simulink model "MSDR_DH_DeplV1sim"  (R2019a)
settings: Solver=ode45  StartTime=0.0  StopTime=simtime  FixedStep=0.1  MaxStep=ts_max  RelTol=rel_tolerance
values from neighbouring files (symbols this model uses):
  a_f = 1E-5*depl_fuel_temp_coef(depl_index)    [MSDR_DH_DeplV1para.m]
  a_g = 1E-5*depl_grap_temp_coef(depl_index)    [MSDR_DH_DeplV1para.m]
  A_s = 1.2245    [MSDR_DH_DeplV1para.m]
  beta = depl_beta(depl_index,:)    [MSDR_DH_DeplV1para.m]
  beta_t = sum(beta)    [MSDR_DH_DeplV1para.m]
  Cp_f = depl_Cp_Fuel_coef*1.355616e-3    [MSDR_DH_DeplV1para.m]
  Cp_p = Cp_s_shx    [MSDR_DH_DeplV1para.m]
  Cp_s = Cp_s*1e-6    (= 3.588208e-09)    [MSDR_DH_DeplV1para.m]
  Cp_sc = 4761.392e-6    (= 0.004761392)    [MSDR_DH_DeplV1para.m]
  Cp_w = 456.056e-6    (= 0.000456056)    [MSDR_DH_DeplV1para.m]
  D_it = 0.0141478    [MSDR_DH_DeplV1para.m]
  D_ot = 0.015875    [MSDR_DH_DeplV1para.m]
  DHRS_TIME_K = 10    [MSDR_DH_DeplV1para.m]
  dHs_dPs = -0.042433622114357    (= -0.0424336221144)    [MSDR_DH_DeplV1para.m]
  Epsilon = 1E-3    (= 0.001)    [MSDR_DH_DeplV1para.m]
  Fiss_factor = 2.464783802008740e-03    (= 0.00246478380201)    [MSDR_DH_DeplV1para.m]
  gamma0 = 9.635981959409105e-01    (= 0.963598195941)    [MSDR_DH_DeplV1para.m]
  gamma1 = 3.560674858154914e-02    (= 0.0356067485815)    [MSDR_DH_DeplV1para.m]
  gamma2 = 7.950554775404400e-04    (= 0.00079505547754)    [MSDR_DH_DeplV1para.m]
  gamma_I = 5.1135e-2    (= 0.051135)    [MSDR_DH_DeplV1para.m]
  gamma_Pm = 1.08E-2    (= 0.0108)    [MSDR_DH_DeplV1para.m]
  gamma_Xe = 1.1628e-2    (= 0.011628)    [MSDR_DH_DeplV1para.m]
  h_pw = h_s_shx    [MSDR_DH_DeplV1para.m]
  h_wb = 13349.334646671E-6    (= 0.0133493346467)    [MSDR_DH_DeplV1para.m]
  h_ws = 5732.378387768E-6    (= 0.00573237838777)    [MSDR_DH_DeplV1para.m]
  h_wsc = 8385.005556375E-6    (= 0.00838500555638)    [MSDR_DH_DeplV1para.m]
  hA_fg = [h_fg*A_fg/2, h_fg*A_fg/2]    [MSDR_DH_DeplV1para.m]
  hA_p_phx1 = h_p_phx*A_p_phx    [MSDR_DH_DeplV1para.m]
  hA_p_phx2 = h_p_phx*A_p_phx    [MSDR_DH_DeplV1para.m]
  hA_p_phx3 = h_p_phx*A_p_phx    [MSDR_DH_DeplV1para.m]
  hA_p_phx4 = h_p_phx*A_p_phx    [MSDR_DH_DeplV1para.m]
  hA_p_phx5 = h_p_phx*A_p_phx    [MSDR_DH_DeplV1para.m]
  hA_p_phx6 = h_p_phx*A_p_phx    [MSDR_DH_DeplV1para.m]
  hA_p_shx1 = h_p_shx*A_p_shx    [MSDR_DH_DeplV1para.m]
  hA_p_shx2 = h_p_shx*A_p_shx    [MSDR_DH_DeplV1para.m]
  hA_p_shx3 = h_p_shx*A_p_shx    [MSDR_DH_DeplV1para.m]
  hA_p_shx4 = h_p_shx*A_p_shx    [MSDR_DH_DeplV1para.m]
  hA_p_shx5 = h_p_shx*A_p_shx    [MSDR_DH_DeplV1para.m]
  hA_p_shx6 = h_p_shx*A_p_shx    [MSDR_DH_DeplV1para.m]
  hA_s_phx1 = h_s_phx*A_s_phx    [MSDR_DH_DeplV1para.m]
  hA_s_phx2 = h_s_phx*A_s_phx    [MSDR_DH_DeplV1para.m]
  hA_s_phx3 = h_s_phx*A_s_phx    [MSDR_DH_DeplV1para.m]
  hA_s_phx4 = h_s_phx*A_s_phx    [MSDR_DH_DeplV1para.m]
  hA_s_phx5 = h_s_phx*A_s_phx    [MSDR_DH_DeplV1para.m]
  hA_s_phx6 = h_s_phx*A_s_phx    [MSDR_DH_DeplV1para.m]
  hA_s_shx1 = h_s_shx*A_s_shx    [MSDR_DH_DeplV1para.m]
  hA_s_shx2 = h_s_shx*A_s_shx    [MSDR_DH_DeplV1para.m]
  hA_s_shx3 = h_s_shx*A_s_shx    [MSDR_DH_DeplV1para.m]
  hA_s_shx4 = h_s_shx*A_s_shx    [MSDR_DH_DeplV1para.m]
  hA_s_shx5 = h_s_shx*A_s_shx    [MSDR_DH_DeplV1para.m]
  hA_s_shx6 = h_s_shx*A_s_shx    [MSDR_DH_DeplV1para.m]
  I_0 = gamma_I*Sig_f_msdr*phi_0/lam_I    [MSDR_DH_DeplV1para.m]
  Ifa = [0.25, 0.25]    [MSDR_DH_DeplV1para.m]
  Ifb = [0.25, 0.25]    [MSDR_DH_DeplV1para.m]
  Ig = [0.5, 0.5]    [MSDR_DH_DeplV1para.m]
  K_1 = 11.632248097704855    (= 11.6322480977)    [MSDR_DH_DeplV1para.m]
  K_4 = b(1)    [MSDR_DH_DeplV1para.m]
  K_5 = a(1)    [MSDR_DH_DeplV1para.m]
  K_b = 12.834854076292217    (= 12.8348540763)    [MSDR_DH_DeplV1para.m]
  K_pump = 1/5    (= 0.2)    [MSDR_DH_DeplV1para.m]
  K_sc = -17.615718797133468    (= -17.6157187971)    [MSDR_DH_DeplV1para.m]
  ka = [0.235, 0.235]    [MSDR_DH_DeplV1para.m]
  kb = [0.235, 0.235]    [MSDR_DH_DeplV1para.m]
  kga = [0.015, 0.015]    [MSDR_DH_DeplV1para.m]
  kgb = [0.015, 0.015]    [MSDR_DH_DeplV1para.m]
  L = 8.5344    [MSDR_DH_DeplV1para.m]
  L_b = 2.3645    [MSDR_DH_DeplV1para.m]
  L_s = 4.723    [MSDR_DH_DeplV1para.m]
  Lam = depl_Lam(depl_index)    [MSDR_DH_DeplV1para.m]
  lam = [1.240E-02, 3.05E-02, 1.11E-01, 3.01E-01, 1.140E+00, 3.014E+00]    [MSDR_DH_DeplV1para.m]
  lam_bubl = 2.0e-2    (= 0.02)    [MSDR_DH_DeplV1para.m]
  lam_I = 2.875e-5    (= 2.875e-05)    [MSDR_DH_DeplV1para.m]
  lam_Pm = log(2)/(2.21*24*3600)    [MSDR_DH_DeplV1para.m]
  lam_Xe = 2.0916e-5    (= 2.0916e-05)    [MSDR_DH_DeplV1para.m]
  lambda0 = 0.0945298    [MSDR_DH_DeplV1para.m]
  lambda1 = 0.00441957    [MSDR_DH_DeplV1para.m]
  lambda2 = 8.60979e-05    [MSDR_DH_DeplV1para.m]
  m_3m = W_3*2    (= 8618.207327)    [MSDR_DH_DeplV1para.m]
  m_f_t = total_mp_phx + core_fm + mp_phxm*3 + m_fm    [MSDR_DH_DeplV1para.m]
  m_fm = W_f*1    (= 4989.48)    [MSDR_DH_DeplV1para.m]
  M_stm = 0.018    [MSDR_DH_DeplV1para.m]
  mcp_fa = mfa*Cp_f    [MSDR_DH_DeplV1para.m]
  mcp_fb = mfb*Cp_f    [MSDR_DH_DeplV1para.m]
  mcp_g = mg*Cp_g    [MSDR_DH_DeplV1para.m]
  mcp_p_phx1 = Cp_p_phx*mp_phx1    [MSDR_DH_DeplV1para.m]
  mcp_p_phx2 = Cp_p_phx*mp_phx2    [MSDR_DH_DeplV1para.m]
  mcp_p_phx3 = Cp_p_phx*mp_phx3    [MSDR_DH_DeplV1para.m]
  mcp_p_phx4 = Cp_p_phx*mp_phx4    [MSDR_DH_DeplV1para.m]
  mcp_p_phx5 = Cp_p_phx*mp_phx5    [MSDR_DH_DeplV1para.m]
  mcp_p_phx6 = Cp_p_phx*mp_phx6    [MSDR_DH_DeplV1para.m]
  mcp_p_shx1 = Cp_p_shx*mp_shx1    [MSDR_DH_DeplV1para.m]
  mcp_p_shx2 = Cp_p_shx*mp_shx2    [MSDR_DH_DeplV1para.m]
  mcp_p_shx3 = Cp_p_shx*mp_shx3    [MSDR_DH_DeplV1para.m]
  mcp_p_shx4 = Cp_p_shx*mp_shx4    [MSDR_DH_DeplV1para.m]
  mcp_p_shx5 = Cp_p_shx*mp_shx5    [MSDR_DH_DeplV1para.m]
  mcp_p_shx6 = Cp_p_shx*mp_shx6    [MSDR_DH_DeplV1para.m]
  mcp_s_phx1 = Cp_s_phx*ms_phx1    [MSDR_DH_DeplV1para.m]
  mcp_s_phx2 = Cp_s_phx*ms_phx2    [MSDR_DH_DeplV1para.m]
  mcp_s_phx3 = Cp_s_phx*ms_phx3    [MSDR_DH_DeplV1para.m]
  mcp_s_phx4 = Cp_s_phx*ms_phx4    [MSDR_DH_DeplV1para.m]
  mcp_s_phx5 = Cp_s_phx*ms_phx5    [MSDR_DH_DeplV1para.m]
  mcp_s_phx6 = Cp_s_phx*ms_phx6    [MSDR_DH_DeplV1para.m]
  mcp_s_shx1 = Cp_s_shx*ms_shx1    [MSDR_DH_DeplV1para.m]
  mcp_s_shx2 = Cp_s_shx*ms_shx1    [MSDR_DH_DeplV1para.m]
  mcp_s_shx3 = Cp_s_shx*ms_shx1    [MSDR_DH_DeplV1para.m]
  mcp_s_shx4 = Cp_s_shx*ms_shx1    [MSDR_DH_DeplV1para.m]
  mcp_s_shx5 = Cp_s_shx*ms_shx1    [MSDR_DH_DeplV1para.m]
  mcp_s_shx6 = Cp_s_shx*ms_shx1    [MSDR_DH_DeplV1para.m]
  mcp_t_phx1 = Cp_t_phx*mt_phx1    [MSDR_DH_DeplV1para.m]
  mcp_t_phx2 = Cp_t_phx*mt_phx2    [MSDR_DH_DeplV1para.m]
  mcp_t_phx3 = Cp_t_phx*mt_phx3    [MSDR_DH_DeplV1para.m]
  mcp_t_phx4 = Cp_t_phx*mt_phx4    [MSDR_DH_DeplV1para.m]
  mcp_t_phx5 = Cp_t_phx*mt_phx5    [MSDR_DH_DeplV1para.m]
  mcp_t_phx6 = Cp_t_phx*mt_phx6    [MSDR_DH_DeplV1para.m]
  mcp_t_shx1 = Cp_t_phx*mt_shx1    [MSDR_DH_DeplV1para.m]
  mcp_t_shx2 = Cp_t_phx*mt_shx2    [MSDR_DH_DeplV1para.m]
  mcp_t_shx3 = Cp_t_phx*mt_shx3    [MSDR_DH_DeplV1para.m]
  mcp_t_shx4 = Cp_t_phx*mt_shx4    [MSDR_DH_DeplV1para.m]
  mcp_t_shx5 = Cp_t_phx*mt_shx5    [MSDR_DH_DeplV1para.m]
  mcp_t_shx6 = Cp_t_phx*mt_shx6    [MSDR_DH_DeplV1para.m]
  ... (+159 more)
undefined symbols (not defined in the file or in its folder): C0, DHRS_MODE, DHRS_Power, DHRS_time, ln, P, Trip_P1_pump, Trip_P2_pump, Trip_P3_pump, Trip_S1_pump, Trip_S2_pump, Trip_S3_pump, Trip_T1_pump, Trip_T2_pump, Trip_T3_pump, Trip_UHX
libraries: simulink x2
(part 3 of 4)

== system MSDR_DH_DeplV1sim/HEAT EXCHANGERS/HEAT EXCHANGER LOOP 3/PHX5 HEAT TRANSFER ==
  PRIMARY FLUID INLET TEMPERATURE : Inport
  SECONDARY FLUID INLET TEMPERATURE : Inport  Port=2
  PRIMARY FLOW FRACTION : Inport  Port=3
  PRIMARY HEAT TRANSFER FRACTION : Inport  Port=4
  SECONDARY FLOW FRACTION : Inport  Port=5
  SECONDARY HEAT TRANSFER FRACTION : Inport  Port=6
  DECAY HEAT : Inport  Port=7
  Mux : Mux  Inputs=17
      settings: DisplayOption=signals
  To Workspace : ToWorkspace  VariableName=phx5_ht  SampleTime=-1
  Tp1_phx5 : Integrator  InitialCondition=T0_p_phx5(1)
  Tp2_phx5 : Integrator  InitialCondition=T0_p_phx5(2)
  "Tp3_phx5 " : Integrator  InitialCondition=T0_p_phx5(3)
  Tp4_phx5 : Integrator  InitialCondition=T0_p_phx5(4)
  Ts1_phx5 : Integrator  InitialCondition=T0_s_phx5(1)
  Ts2_phx5 : Integrator  InitialCondition=T0_s_phx5(2)
  Ts3_phx5 : Integrator  InitialCondition=T0_s_phx5(3)
  Ts4_phx5 : Integrator  InitialCondition=T0_s_phx5(4)
  Tt1_phx5 : Integrator  InitialCondition=T0_t_phx5(1)
  Tt2_phx5 : Integrator  InitialCondition=T0_t_phx5(2)
  d(Tp1_phx5)/dt : Fcn  Expr=(u[13]*Wp_phx5/mp_phx5(1))*(u[1] - u[3]) + (u[14]*hA_p_phx5(1)/mcp_p_phx5(1))*(u[7] - u[3]) + u(17)*P*mp_phx5(1)/(m_f_t*mcp_p_phx5(1))
  d(Tp2_phx5)/dt : Fcn  Expr=(u[13]*Wp_phx5/mp_phx5(2))*(u[3] - u[4]) + (u[14]*hA_p_phx5(2)/mcp_p_phx5(2))*(u[7] - u[3]) + u(17)*P*mp_phx5(2)/(m_f_t*mcp_p_phx5(2))
  d(Tp3_phx5)/dt : Fcn  Expr=(u[13]*Wp_phx5/mp_phx5(3))*(u[4] - u[5]) + (u[14]*hA_p_phx5(3)/mcp_p_phx5(3))*(u[8] - u[5]) + u(17)*P*mp_phx5(3)/(m_f_t*mcp_p_phx5(3))
  d(Tp4_phx5)/dt : Fcn  Expr=(u[13]*Wp_phx5/mp_phx5(4))*(u[5] - u[6]) + (u[14]*hA_p_phx5(4)/mcp_p_phx5(4))*(u[8] - u[5]) + u(17)*P*mp_phx5(4)/(m_f_t*mcp_p_phx5(4))
  d(Ts1_phx5)/dt : Fcn  Expr=(u[15]*Ws_phx5/ms_phx5(1))*(u[2] - u[9]) + (u[16]*hA_s_phx5(1)/mcp_s_phx5(1))*(u[8] - u[9])
  d(Ts2_phx5)/dt : Fcn  Expr=(u[15]*Ws_phx5/ms_phx5(2))*(u[9] - u[10]) + (u[16]*hA_s_phx5(2)/mcp_s_phx5(2))*(u[8] - u[9])
  d(Ts3_phx5)/dt : Fcn  Expr=(u[15]*Ws_phx5/ms_phx5(3))*(u[10] - u[11]) + (u[16]*hA_s_phx5(3)/mcp_s_phx5(3))*(u[7] - u[11])
  d(Ts4_phx5)/dt : Fcn  Expr=(u[15]*Ws_phx5/ms_phx5(4))*(u[11] - u[12]) + (u[16]*hA_s_phx5(4)/mcp_s_phx5(4))*(u[7] - u[11])
  d(Tt1_phx3)/dt : Fcn  Expr=(u[14]*(hA_p_phx5(1) + hA_p_phx5(2))/mcp_t_phx5(1))*(u[3] - u[7]) + (u[16]*(hA_s_phx5(1) + hA_s_phx5(2))/mcp_t_phx5(1))*(u[11] - u[7])
  d(Tt2_phx5)/dt : Fcn  Expr=(u[14]*(hA_p_phx5(3) + hA_p_phx5(4))/mcp_t_phx5(2))*(u[5] - u[8]) + (u[16]*(hA_s_phx5(3) + hA_s_phx5(4))/mcp_t_phx5(2))*(u[9] - u[8])
  PHX5 TEMPERATURES : Outport
  wires:
  Ts1_phx5/1 -> Mux/9
  Ts2_phx5/1 -> Mux/10
  d(Ts2_phx5)/dt/1 -> Ts2_phx5/1
  d(Tp4_phx5)/dt/1 -> Tp4_phx5/1
  Tt1_phx5/1 -> Mux/7
  d(Tp2_phx5)/dt/1 -> Tp2_phx5/1
  Tp4_phx5/1 -> Mux/6
  d(Tt2_phx5)/dt/1 -> Tt2_phx5/1
  SECONDARY FLUID INLET TEMPERATURE/1 -> Mux/2
  Tt2_phx5/1 -> Mux/8
  Mux/1 -> To Workspace/1, PHX5 TEMPERATURES/1, d(Ts4_phx5)/dt/1, d(Ts3_phx5)/dt/1, d(Ts1_phx5)/dt/1, d(Tt2_phx5)/dt/1, d(Tt1_phx3)/dt/1, d(Tp4_phx5)/dt/1, d(Tp3_phx5)/dt/1, d(Tp2_phx5)/dt/1, d(Tp1_phx5)/dt/1, d(Ts2_phx5)/dt/1
  d(Tp1_phx5)/dt/1 -> Tp1_phx5/1
  d(Ts4_phx5)/dt/1 -> Ts4_phx5/1
  Tp1_phx5/1 -> Mux/3
  d(Ts1_phx5)/dt/1 -> Ts1_phx5/1
  d(Ts3_phx5)/dt/1 -> Ts3_phx5/1
  Ts3_phx5/1 -> Mux/11
  Ts4_phx5/1 -> Mux/12
  "Tp3_phx5 "/1 -> Mux/5
  d(Tp3_phx5)/dt/1 -> "Tp3_phx5 "/1
  Tp2_phx5/1 -> Mux/4
  d(Tt1_phx3)/dt/1 -> Tt1_phx5/1
  PRIMARY FLUID INLET TEMPERATURE/1 -> Mux/1
  PRIMARY FLOW FRACTION/1 -> Mux/13
  PRIMARY HEAT TRANSFER FRACTION/1 -> Mux/14
  SECONDARY FLOW FRACTION/1 -> Mux/15
  SECONDARY HEAT TRANSFER FRACTION/1 -> Mux/16
  DECAY HEAT/1 -> Mux/17

== system MSDR_DH_DeplV1sim/HEAT EXCHANGERS/HEAT EXCHANGER LOOP 3/PHX6 HEAT TRANSFER ==
  PRIMARY FLUID INLET TEMPERATURE : Inport
  SECONDARY FLUID INLET TEMPERATURE : Inport  Port=2
  PRIMARY FLOW FRACTION : Inport  Port=3
  PRIMARY HEAT TRANSFER FRACTION : Inport  Port=4
  SECONDARY FLOW FRACTION : Inport  Port=5
  SECONDARY HEAT TRANSFER FRACTION : Inport  Port=6
  DECAY HEAT : Inport  Port=7
  Mux : Mux  Inputs=17
      settings: DisplayOption=signals
  To Workspace : ToWorkspace  VariableName=phx6_ht  SampleTime=-1
  Tp1_phx6 : Integrator  InitialCondition=T0_p_phx6(1)
  Tp2_phx6 : Integrator  InitialCondition=T0_p_phx6(2)
  "Tp3_phx6 " : Integrator  InitialCondition=T0_p_phx6(3)
  Tp4_phx6 : Integrator  InitialCondition=T0_p_phx6(4)
  Ts1_phx6 : Integrator  InitialCondition=T0_s_phx6(1)
  Ts2_phx6 : Integrator  InitialCondition=T0_s_phx6(2)
  Ts3_phx6 : Integrator  InitialCondition=T0_s_phx6(3)
  Ts4_phx6 : Integrator  InitialCondition=T0_s_phx6(4)
  Tt1_phx6 : Integrator  InitialCondition=T0_t_phx6(1)
  Tt2_phx6 : Integrator  InitialCondition=T0_t_phx6(2)
  d(Tp1_phx6)/dt : Fcn  Expr=(u[13]*Wp_phx6/mp_phx6(1))*(u[1] - u[3]) + (u[14]*hA_p_phx6(1)/mcp_p_phx6(1))*(u[7] - u[3]) + u(17)*P*mp_phx6(1)/(m_f_t*mcp_p_phx6(1))
  d(Tp2_phx6)/dt : Fcn  Expr=(u[13]*Wp_phx6/mp_phx6(2))*(u[3] - u[4]) + (u[14]*hA_p_phx6(2)/mcp_p_phx6(2))*(u[7] - u[3]) + u(17)*P*mp_phx6(2)/(m_f_t*mcp_p_phx6(2))
  d(Tp3_phx6)/dt : Fcn  Expr=(u[13]*Wp_phx6/mp_phx6(3))*(u[4] - u[5]) + (u[14]*hA_p_phx6(3)/mcp_p_phx6(3))*(u[8] - u[5]) + u(17)*P*mp_phx6(3)/(m_f_t*mcp_p_phx6(3))
  d(Tp4_phx6)/dt : Fcn  Expr=(u[13]*Wp_phx6/mp_phx6(4))*(u[5] - u[6]) + (u[14]*hA_p_phx6(4)/mcp_p_phx6(4))*(u[8] - u[5]) + u(17)*P*mp_phx6(4)/(m_f_t*mcp_p_phx6(4))
  d(Ts1_phx6)/dt : Fcn  Expr=(u[15]*Ws_phx6/ms_phx6(1))*(u[2] - u[9]) + (u[16]*hA_s_phx6(1)/mcp_s_phx6(1))*(u[8] - u[9])
  d(Ts2_phx6)/dt : Fcn  Expr=(u[15]*Ws_phx6/ms_phx6(2))*(u[9] - u[10]) + (u[16]*hA_s_phx6(2)/mcp_s_phx6(2))*(u[8] - u[9])
  d(Ts3_phx6)/dt : Fcn  Expr=(u[15]*Ws_phx6/ms_phx6(3))*(u[10] - u[11]) + (u[16]*hA_s_phx6(3)/mcp_s_phx6(3))*(u[7] - u[11])
  d(Ts4_phx6)/dt : Fcn  Expr=(u[15]*Ws_phx6/ms_phx6(4))*(u[11] - u[12]) + (u[16]*hA_s_phx6(4)/mcp_s_phx6(4))*(u[7] - u[11])
  d(Tt1_phx6)/dt : Fcn  Expr=(u[14]*(hA_p_phx6(1) + hA_p_phx6(2))/mcp_t_phx6(1))*(u[3] - u[7]) + (u[16]*(hA_s_phx6(1) + hA_s_phx6(2))/mcp_t_phx6(1))*(u[11] - u[7])
  d(Tt2_phx6)/dt : Fcn  Expr=(u[14]*(hA_p_phx6(3) + hA_p_phx6(4))/mcp_t_phx6(2))*(u[5] - u[8]) + (u[16]*(hA_s_phx6(3) + hA_s_phx6(4))/mcp_t_phx6(2))*(u[9] - u[8])
  PHX6 TEMPERATURES : Outport
  wires:
  Ts1_phx6/1 -> Mux/9
  Ts2_phx6/1 -> Mux/10
  d(Ts2_phx6)/dt/1 -> Ts2_phx6/1
  d(Tp4_phx6)/dt/1 -> Tp4_phx6/1
  Tt1_phx6/1 -> Mux/7
  d(Tp2_phx6)/dt/1 -> Tp2_phx6/1
  Tp4_phx6/1 -> Mux/6
  d(Tt2_phx6)/dt/1 -> Tt2_phx6/1
  SECONDARY FLUID INLET TEMPERATURE/1 -> Mux/2
  Tt2_phx6/1 -> Mux/8
  Mux/1 -> To Workspace/1, PHX6 TEMPERATURES/1, d(Ts4_phx6)/dt/1, d(Ts3_phx6)/dt/1, d(Ts1_phx6)/dt/1, d(Tt2_phx6)/dt/1, d(Tt1_phx6)/dt/1, d(Tp4_phx6)/dt/1, d(Tp3_phx6)/dt/1, d(Tp2_phx6)/dt/1, d(Tp1_phx6)/dt/1, d(Ts2_phx6)/dt/1
  d(Tp1_phx6)/dt/1 -> Tp1_phx6/1
  d(Ts4_phx6)/dt/1 -> Ts4_phx6/1
  Tp1_phx6/1 -> Mux/3
  d(Ts1_phx6)/dt/1 -> Ts1_phx6/1
  d(Ts3_phx6)/dt/1 -> Ts3_phx6/1
  Ts3_phx6/1 -> Mux/11
  Ts4_phx6/1 -> Mux/12
  "Tp3_phx6 "/1 -> Mux/5
  d(Tp3_phx6)/dt/1 -> "Tp3_phx6 "/1
  Tp2_phx6/1 -> Mux/4
  d(Tt1_phx6)/dt/1 -> Tt1_phx6/1
  PRIMARY FLUID INLET TEMPERATURE/1 -> Mux/1
  SECONDARY FLOW FRACTION/1 -> Mux/15
  PRIMARY HEAT TRANSFER FRACTION/1 -> Mux/14
  PRIMARY FLOW FRACTION/1 -> Mux/13
  SECONDARY HEAT TRANSFER FRACTION/1 -> Mux/16
  DECAY HEAT/1 -> Mux/17

== system MSDR_DH_DeplV1sim/HEAT EXCHANGERS/HEAT EXCHANGER LOOP 3/SHX PRIM MIXING ==
  Tp_shx5 : Inport
  Tp_shx6 : Inport  Port=2
  p_flow_frac : Inport  Port=3
  Fcn : Fcn  Expr=u[3]*Wp_shx5/mp_shxm*(u[1]-u[4]) + u[3]*Wp_shx6/mp_shxm*(u[2]-u[4])
  Integrator : Integrator  InitialCondition=T0_p_shx1(4)
  Mux : Mux
  Tp_shx_mix : Outport
  wires:
  Tp_shx5/1 -> Mux/1
  Tp_shx6/1 -> Mux/2
  Mux/1 -> Fcn/1
  p_flow_frac/1 -> Mux/3
  Fcn/1 -> Integrator/1
  Integrator/1 -> Tp_shx_mix/1, Mux/4

== system MSDR_DH_DeplV1sim/HEAT EXCHANGERS/HEAT EXCHANGER LOOP 3/SHX SEC MIXING ==
  Ts_shx5 : Inport
  Ts_shx6 : Inport  Port=2
  s_flow_frac : Inport  Port=3
  Fcn : Fcn  Expr=u[3]*Ws_shx5/ms_shxm*(u[1]-u[4]) + u[3]*Ws_shx6/ms_shxm*(u[2]-u[4])
  Integrator : Integrator  InitialCondition=T0_s_shx1(4)
  Mux : Mux
  Ts_shx_mix : Outport
  wires:
  Ts_shx5/1 -> Mux/1
  Ts_shx6/1 -> Mux/2
  Mux/1 -> Fcn/1
  s_flow_frac/1 -> Mux/3
  Fcn/1 -> Integrator/1
  Integrator/1 -> Ts_shx_mix/1, Mux/4

== system MSDR_DH_DeplV1sim/HEAT EXCHANGERS/HEAT EXCHANGER LOOP 3/SHX//THX PUMP ==
  Clock1 : Clock
  Fcn1 : Fcn  Expr=(1-therm_conv)*exp(-K_pump*(u))+therm_conv
  H.T.C. as f(flow_fraction) : Fcn  Expr=0.8215*u^6-4.108*u^5+7.848*u^4-7.165*u^3+3.004*u^2+0.5903*u+0.008537
  Pump Trip Time : TransportDelay  DelayTime=Trip_T3_pump  BufferSize=4096
  FLOW FRACTION : Outport
  HEAT TRANSFER FRACTION : Outport  Port=2
  wires:
  H.T.C. as f(flow_fraction)/1 -> HEAT TRANSFER FRACTION/1
  Clock1/1 -> Pump Trip Time/1
  Pump Trip Time/1 -> Fcn1/1
  Fcn1/1 -> FLOW FRACTION/1, H.T.C. as f(flow_fraction)/1

== system MSDR_DH_DeplV1sim/HEAT EXCHANGERS/HEAT EXCHANGER LOOP 3/SHX5 HEAT TRANSFER ==
  PRIMARY FLUID INLET TEMPERATURE : Inport
  SECONDARY FLUID INLET TEMPERATURE : Inport  Port=2
  PRIMARY FLOW FRACTION : Inport  Port=3
  PRIMARY HEAT TRANSFER FRACTION : Inport  Port=4
  SECONDARY FLOW FRACTION : Inport  Port=5
  SECONDARY HEAT TRANSFER FRACTION : Inport  Port=6
  Mux : Mux  Inputs=16
      settings: DisplayOption=signals
  To Workspace : ToWorkspace  VariableName=shx5_ht  SampleTime=-1
  Tp1_shx5 : Integrator  InitialCondition=T0_p_shx3(1)
  Tp2_shx5 : Integrator  InitialCondition=T0_p_shx5(2)
  "Tp3_shx5 " : Integrator  InitialCondition=T0_p_shx5(3)
  Tp4_shx5 : Integrator  InitialCondition=T0_p_shx5(4)
  Ts1_shx5 : Integrator  InitialCondition=T0_s_shx5(1)
  Ts2_shx5 : Integrator  InitialCondition=T0_s_shx5(2)
  Ts3_shx5 : Integrator  InitialCondition=T0_s_shx5(3)
  Ts4_shx5 : Integrator  InitialCondition=T0_s_shx5(4)
  Tt1_shx5 : Integrator  InitialCondition=T0_t_shx5(1)
  Tt2_shx5 : Integrator  InitialCondition=T0_t_shx5(2)
  d(Tp1_shx5)/dt : Fcn  Expr=(u[13]*Wp_shx5/mp_shx5(1))*(u[1] - u[3]) + (u[14]*hA_p_shx5(1)/mcp_p_shx5(1))*(u[7] - u[3])
  d(Tp2_shx5)/dt : Fcn  Expr=(u[13]*Wp_shx5/mp_shx5(2))*(u[3] - u[4]) + (u[14]*hA_p_shx5(2)/mcp_p_shx5(2))*(u[7] - u[3])
  d(Tp3_shx5)/dt : Fcn  Expr=(u[13]*Wp_shx5/mp_shx5(3))*(u[4] - u[5]) + (u[14]*hA_p_shx5(3)/mcp_p_shx5(3))*(u[8] - u[5])
  d(Tp4_shx5)/dt : Fcn  Expr=(u[13]*Wp_shx5/mp_shx5(4))*(u[5] - u[6]) + (u[14]*hA_p_shx5(4)/mcp_p_shx5(4))*(u[8] - u[5])
  d(Ts1_shx5)/dt : Fcn  Expr=(u[15]*Ws_shx5/ms_shx5(1))*(u[2] - u[9]) + (u[16]*hA_s_shx5(1)/mcp_s_shx5(1))*(u[8] - u[9])
  d(Ts2_shx5)/dt : Fcn  Expr=(u[15]*Ws_shx5/ms_shx5(2))*(u[9] - u[10]) + (u[16]*hA_s_shx5(2)/mcp_s_shx5(2))*(u[8] - u[9])
  d(Ts3_shx5)/dt : Fcn  Expr=(u[15]*Ws_shx5/ms_shx5(3))*(u[10] - u[11]) + (u[16]*hA_s_shx5(3)/mcp_s_shx5(3))*(u[7] - u[11])
  d(Ts4_shx5)/dt : Fcn  Expr=(u[15]*Ws_shx5/ms_shx5(4))*(u[11] - u[12]) + (u[16]*hA_s_shx5(4)/mcp_s_shx5(4))*(u[7] - u[11])
  d(Tt1_shx5)/dt : Fcn  Expr=(u[14]*(hA_p_shx5(1) + hA_p_shx5(2))/mcp_t_shx5(1))*(u[3] - u[7]) + (u[16]*(hA_s_shx5(1) + hA_s_shx5(2))/mcp_t_shx5(1))*(u[11] - u[7])
  d(Tt2_shx5)/dt : Fcn  Expr=(u[14]*(hA_p_shx5(3) + hA_p_shx5(4))/mcp_t_shx5(2))*(u[5] - u[8]) + (u[16]*(hA_s_shx5(3) + hA_s_shx5(4))/mcp_t_shx5(2))*(u[9] - u[8])
  SHX5 TEMPERATURES : Outport
  wires:
  Ts1_shx5/1 -> Mux/9
  Ts2_shx5/1 -> Mux/10
  d(Ts2_shx5)/dt/1 -> Ts2_shx5/1
  d(Tp4_shx5)/dt/1 -> Tp4_shx5/1
  Tt1_shx5/1 -> Mux/7
  d(Tp2_shx5)/dt/1 -> Tp2_shx5/1
  Tp4_shx5/1 -> Mux/6
  d(Tt2_shx5)/dt/1 -> Tt2_shx5/1
  SECONDARY FLUID INLET TEMPERATURE/1 -> Mux/2
  Tt2_shx5/1 -> Mux/8
  Mux/1 -> To Workspace/1, SHX5 TEMPERATURES/1, d(Ts4_shx5)/dt/1, d(Ts3_shx5)/dt/1, d(Ts2_shx5)/dt/1, d(Ts1_shx5)/dt/1, d(Tt2_shx5)/dt/1, d(Tt1_shx5)/dt/1, d(Tp4_shx5)/dt/1, d(Tp3_shx5)/dt/1, d(Tp2_shx5)/dt/1, d(Tp1_shx5)/dt/1
  d(Tp1_shx5)/dt/1 -> Tp1_shx5/1
  d(Ts4_shx5)/dt/1 -> Ts4_shx5/1
  Tp1_shx5/1 -> Mux/3
  d(Ts1_shx5)/dt/1 -> Ts1_shx5/1
  d(Ts3_shx5)/dt/1 -> Ts3_shx5/1
  Ts3_shx5/1 -> Mux/11
  Ts4_shx5/1 -> Mux/12
  "Tp3_shx5 "/1 -> Mux/5
  d(Tp3_shx5)/dt/1 -> "Tp3_shx5 "/1
  Tp2_shx5/1 -> Mux/4
  d(Tt1_shx5)/dt/1 -> Tt1_shx5/1
  PRIMARY FLUID INLET TEMPERATURE/1 -> Mux/1
  SECONDARY FLOW FRACTION/1 -> Mux/15
  PRIMARY HEAT TRANSFER FRACTION/1 -> Mux/14
  PRIMARY FLOW FRACTION/1 -> Mux/13
  SECONDARY HEAT TRANSFER FRACTION/1 -> Mux/16

== system MSDR_DH_DeplV1sim/HEAT EXCHANGERS/HEAT EXCHANGER LOOP 3/SHX6 HEAT TRANSFER ==
  PRIMARY FLUID INLET TEMPERATURE : Inport
  SECONDARY FLUID INLET TEMPERATURE : Inport  Port=2
  PRIMARY FLOW FRACTION : Inport  Port=3
  PRIMARY HEAT TRANSFER FRACTION : Inport  Port=4
  SECONDARY FLOW FRACTION : Inport  Port=5
  SECONDARY HEAT TRANSFER FRACTION : Inport  Port=6
  Mux : Mux  Inputs=16
      settings: DisplayOption=signals
  To Workspace : ToWorkspace  VariableName=shx6_ht  SampleTime=-1
  Tp1_shx6 : Integrator  InitialCondition=T0_p_shx6(1)
  Tp2_shx6 : Integrator  InitialCondition=T0_p_shx6(2)
  "Tp3_shx6 " : Integrator  InitialCondition=T0_p_shx6(3)
  Tp4_shx6 : Integrator  InitialCondition=T0_p_shx6(4)
  Ts1_shx6 : Integrator  InitialCondition=T0_s_shx6(1)
  Ts2_shx6 : Integrator  InitialCondition=T0_s_shx6(2)
  Ts3_shx6 : Integrator  InitialCondition=T0_s_shx6(3)
  Ts4_shx6 : Integrator  InitialCondition=T0_s_shx6(4)
  Tt1_shx6 : Integrator  InitialCondition=T0_t_shx6(1)
  Tt2_shx6 : Integrator  InitialCondition=T0_t_shx6(2)
  d(Tp1_shx6)/dt : Fcn  Expr=(u[13]*Wp_shx6/mp_shx6(1))*(u[1] - u[3]) + (u[14]*hA_p_shx6(1)/mcp_p_shx6(1))*(u[7] - u[3])
  d(Tp2_shx6)/dt : Fcn  Expr=(u[13]*Wp_shx6/mp_shx6(2))*(u[3] - u[4]) + (u[14]*hA_p_shx6(2)/mcp_p_shx6(2))*(u[7] - u[3])
  d(Tp3_shx6)/dt : Fcn  Expr=(u[13]*Wp_shx6/mp_shx6(3))*(u[4] - u[5]) + (u[14]*hA_p_shx6(3)/mcp_p_shx6(3))*(u[8] - u[5])
  d(Tp4_shx6)/dt : Fcn  Expr=(u[13]*Wp_shx6/mp_shx6(4))*(u[5] - u[6]) + (u[14]*hA_p_shx6(4)/mcp_p_shx6(4))*(u[8] - u[5])
  d(Ts1_shx6)/dt : Fcn  Expr=(u[15]*Ws_shx6/ms_shx6(1))*(u[2] - u[9]) + (u[16]*hA_s_shx6(1)/mcp_s_shx6(1))*(u[8] - u[9])
  d(Ts2_shx6)/dt : Fcn  Expr=(u[15]*Ws_shx6/ms_shx6(2))*(u[9] - u[10]) + (u[16]*hA_s_shx6(2)/mcp_s_shx6(2))*(u[8] - u[9])
  d(Ts3_shx6)/dt : Fcn  Expr=(u[15]*Ws_shx6/ms_shx6(3))*(u[10] - u[11]) + (u[16]*hA_s_shx6(3)/mcp_s_shx6(3))*(u[7] - u[11])
  d(Ts4_shx4)/dt : Fcn  Expr=(u[15]*Ws_shx6/ms_shx6(4))*(u[11] - u[12]) + (u[16]*hA_s_shx6(4)/mcp_s_shx6(4))*(u[7] - u[11])
  d(Tt1_shx6)/dt : Fcn  Expr=(u[14]*(hA_p_shx6(1) + hA_p_shx6(2))/mcp_t_shx6(1))*(u[3] - u[7]) + (u[16]*(hA_s_shx6(1) + hA_s_shx6(2))/mcp_t_shx6(1))*(u[11] - u[7])
  d(Tt2_shx6)/dt : Fcn  Expr=(u[14]*(hA_p_shx6(3) + hA_p_shx6(4))/mcp_t_shx6(2))*(u[5] - u[8]) + (u[16]*(hA_s_shx6(3) + hA_s_shx6(4))/mcp_t_shx6(2))*(u[9] - u[8])
  SHX6 TEMPERATURES : Outport
  wires:
  Ts1_shx6/1 -> Mux/9
  Ts2_shx6/1 -> Mux/10
  d(Ts2_shx6)/dt/1 -> Ts2_shx6/1
  d(Tp4_shx6)/dt/1 -> Tp4_shx6/1
  Tt1_shx6/1 -> Mux/7
  d(Tp2_shx6)/dt/1 -> Tp2_shx6/1
  Tp4_shx6/1 -> Mux/6
  d(Tt2_shx6)/dt/1 -> Tt2_shx6/1
  SECONDARY FLUID INLET TEMPERATURE/1 -> Mux/2
  Tt2_shx6/1 -> Mux/8
  Mux/1 -> To Workspace/1, SHX6 TEMPERATURES/1, d(Ts4_shx4)/dt/1, d(Ts3_shx6)/dt/1, d(Ts2_shx6)/dt/1, d(Ts1_shx6)/dt/1, d(Tt2_shx6)/dt/1, d(Tt1_shx6)/dt/1, d(Tp4_shx6)/dt/1, d(Tp3_shx6)/dt/1, d(Tp2_shx6)/dt/1, d(Tp1_shx6)/dt/1
  d(Tp1_shx6)/dt/1 -> Tp1_shx6/1
  d(Ts4_shx4)/dt/1 -> Ts4_shx6/1
  Tp1_shx6/1 -> Mux/3
  d(Ts1_shx6)/dt/1 -> Ts1_shx6/1
  d(Ts3_shx6)/dt/1 -> Ts3_shx6/1
  Ts3_shx6/1 -> Mux/11
  Ts4_shx6/1 -> Mux/12
  "Tp3_shx6 "/1 -> Mux/5
  d(Tp3_shx6)/dt/1 -> "Tp3_shx6 "/1
  Tp2_shx6/1 -> Mux/4
  d(Tt1_shx6)/dt/1 -> Tt1_shx6/1
  PRIMARY FLUID INLET TEMPERATURE/1 -> Mux/1
  SECONDARY FLOW FRACTION/1 -> Mux/15
  PRIMARY HEAT TRANSFER FRACTION/1 -> Mux/14
  PRIMARY FLOW FRACTION/1 -> Mux/13
  SECONDARY HEAT TRANSFER FRACTION/1 -> Mux/16

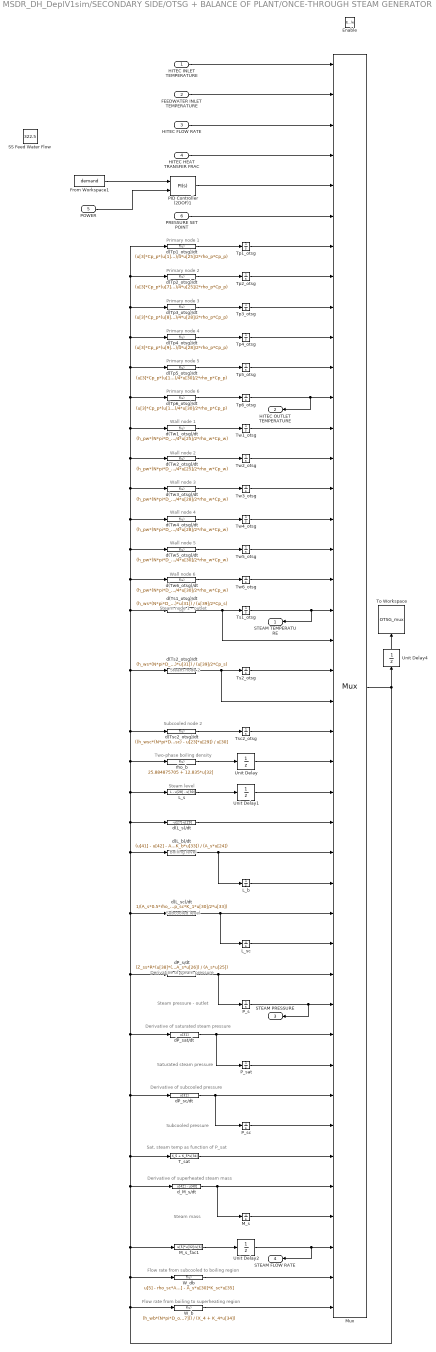
== system MSDR_DH_DeplV1sim/SECONDARY SIDE/OTSG + BALANCE OF PLANT/ONCE-THROUGH STEAM GENERATOR ==
  note: Primary node 1
  note: Primary node 2
  note: Primary node 3
  note: Primary node 4
  note: Primary node 5
  note: Primary node 6
  note: Wall node 1
  note: Wall node 2
  note: Wall node 3
  note: Wall node 4
  note: Wall node 5
  note: Wall node 6
  note: Steam node 1 - outlet
  note: Steam level
  note: Boiling level
  note: Subcooled level
  note: Derivative of saturated steam pressure
  note: Sat. steam temp as function of P_sat
  note: Saturated steam pressure
  note: Subcooled pressure
  note: Derivative of steam pressure
  note: Derivative of subcooled pressure
  note: Steam pressure - outlet
  note: Subcooled node 2
  note: Steam node 2
  note: Two-phase boiling density
  note: Derivative of superheated steam mass
  note: Steam mass
  note: Flow rate from subcooled to boiling region
  note: Flow rate from boiling to superheating region
  HITEC INLET TEMPERATURE : Inport
  FEEDWATER INLET TEMPERATURE : Inport  Port=2
  HITEC FLOW RATE : Inport  Port=3
  HITEC HEAT TRANSFER FRAC : Inport  Port=4
  POWER : Inport  Port=5
  PRESSURE SET POINT : Inport  Port=6
  Enable : EnablePort
  From Workspace1 : FromWorkspace  VariableName=demand  SampleTime=1  Interpolate=off  OutputAfterFinalValue=Holding final value
  L_b : Integrator  InitialCondition=L_b
  L_s : Fcn  Expr=L - u[28] - u[30]
  L_sc : Integrator  InitialCondition=.5344
  M_s : Integrator  InitialCondition=A_s*rho_s*L_s
  M_s_fac1 : Fcn  Expr=u[5]*u[32]/u[6]
  Mux : Mux  Inputs=42
      settings: DisplayOption=signals
  PID Controller (2DOF)1 : simulink/Continuous/PID Controller (2DOF)  Controller=PI  Form=Parallel  TimeDomain=Continuous-time  SampleTime=-1  IntegratorMethod=Forward Euler  FilterMethod=Forward Euler  ControllerParametersSource=internal  P=250  I=5  D=1  UseFilter=on  N=100  b=1  c=1  TunerSelectOption=Transfer Function Based (PID Tuner App)  InitialConditionSource=internal  InitialConditionForIntegrator=0  InitialConditionForFilter=0  DifferentiatorICPrevScaledInput=0  ExternalReset=none  TrackingMode=off  Kt=1  LimitOutput=on  UpperSaturationLimit=1000000  LowerSaturationLimit=1  LinearizeAsGain=on  AntiWindupMode=none  Kb=1  POutMin=[]  POutMax=[]  IOutMin=[]  IOutMax=[]  DOutMin=[]  DOutMax=[]  NOutMin=[]  NOutMax=[]  bOutMin=[]  bOutMax=[]  cOutMin=[]  cOutMax=[]  SumOutMin=[]  SumOutMax=[]  SaturationOutMin=[]  SaturationOutMax=[]  PParamMin=[]  PParamMax=[]  IParamMin=[]  IParamMax=[]  DParamMin=[]  DParamMax=[]  NParamMin=[]  NParamMax=[]  bParamMin=[]  bParamMax=[]  cParamMin=[]  cParamMax=[]  KbParamMin=[]  KbParamMax=[]  KtParamMin=[]  KtParamMax=[]  KbOutMin=[]  KbOutMax=[]  KtOutMin=[]  KtOutMax=[]  IntegratorOutMin=[]  IntegratorOutMax=[]  FilterOutMin=[]  FilterOutMax=[]  SumI1OutMin=[]  SumI1OutMax=[]  SumI2OutMin=[]  SumI2OutMax=[]  SumI3OutMin=[]  SumI3OutMax=[]  SumI4OutMin=[]  SumI4OutMax=[]  SumDOutMin=[]  SumDOutMax=[]  Sum1OutMin=[]  Sum1OutMax=[]  Sum2OutMin=[]  Sum2OutMax=[]  Sum3OutMin=[]  Sum3OutMax=[]  DifferentiatorOutMin=[]  DifferentiatorOutMax=[]  FilterDiffOutCoefMin=[]  FilterDiffOutCoefMax=[]  ReciprocalOutMin=[]  ReciprocalOutMax=[]  SumDenOutMin=[]  SumDenOutMax=[]  SumNumOutMin=[]  SumNumOutMax=[]  DivideOutMin=[]  DivideOutMax=[]  IntegratorContinuousStateAttributes=''  IntegratorStateMustResolveToSignalObject=off  IntegratorRTWStateStorageClass=Auto  FilterContinuousStateAttributes=''  FilterStateMustResolveToSignalObject=off  FilterRTWStateStorageClass=Auto  ParallelPVariant=InternalParameters  IdealPVariant=Disabled  IVariant=InternalParameters  DVariant=Disabled  bVariant=InternalParameters  cVariant=Disabled  IntegratorVariant=Continuous  SatVariant=Enabled  AWVariant=Passthrough  PCopyVariant=Disabled  TRVariant=Disabled  FdbkBlocksVariant=Forward  IdealPFdbkVariant=Disabled  SatFdbkVariant=Disabled  DerivativeFilterVariant=Disabled  NVariant=Disabled  NCopyVariant=Disabled_SignalSpec  FilterICVariant=Disabled  IntegratorICVariant=InternalICs  ExternalResetVariant=Disabled  TRSumVariant=Passthrough  SumFdbkVariant=Disabled  SumVariant=Sum_PI
  P_s : Integrator  InitialCondition=P_s
  P_sat : Integrator  InitialCondition=P_sat
  P_sc : Integrator  InitialCondition=P_sc
  SS Feed Water Flow : Constant  Value=322.5
  T_sat : Fcn  Expr=X_5 + K_5*u[34]
  To Workspace : ToWorkspace  VariableName=OTSG_mux  SaveFormat=Timeseries  SampleTime=-1
  Tp1_otsg : Integrator  InitialCondition=T_p1
  Tp2_otsg : Integrator  InitialCondition=T_p2
  Tp3_otsg : Integrator  InitialCondition=T_p3
  Tp4_otsg : Integrator  InitialCondition=T_p4
  Tp5_otsg : Integrator  InitialCondition=T_p5
  Tp6_otsg : Integrator  InitialCondition=T_p6
  Ts1_otsg : Integrator  InitialCondition=T_s1
  Ts2_otsg : Integrator  InitialCondition=T_s2
  Tsc2_otsg : Integrator  InitialCondition=T_sc2
  Tw1_otsg : Integrator  InitialCondition=T_w1
  Tw2_otsg : Integrator  InitialCondition=T_w2
  Tw3_otsg : Integrator  InitialCondition=T_w3
  Tw4_otsg : Integrator  InitialCondition=T_w4
  Tw5_otsg : Integrator  InitialCondition=T_w5
  Tw6_otsg : Integrator  InitialCondition=T_w6
  Unit Delay : UnitDelay  InitialCondition=rho_b  SampleTime=-1  HasFrameUpgradeWarning=on
  Unit Delay1 : UnitDelay  InitialCondition=L_s  SampleTime=-1  HasFrameUpgradeWarning=on
  Unit Delay2 : UnitDelay  InitialCondition=W_fw  SampleTime=-1  HasFrameUpgradeWarning=on
  Unit Delay4 : UnitDelay  SampleTime=-1  HasFrameUpgradeWarning=on
  W_b : Fcn  Expr=(h_wb*(N*pi*D_ot*u[28])*(0.5*u[15] + 0.5*u[16] - u[37])) / (X_4 + K_4*u[34])
  W_db : Fcn  Expr=u[5] - rho_sc*A_s*u[29] - A_s*u[30]*K_sc*u[35]
  d(L_b)/dt : Fcn  Expr=(u[41] - u[42] - A_s*u[28]*K_b*u[33]) / (A_s*u[24])
  d(L_s)/dt : Fcn  Expr=-u[27]-u[29]
  d(L_sc)/dt : Fcn  Expr=1/(A_s*0.5*rho_sc*Cp_sc*(u[23] - u[37])) * (h_wsc*N*pi*D_ot*u[30]/2*(u[17] - u[37]) + Cp_sc*(u[5]*u[23] - (u[5] + u[41])*0.5*u[37]) - A_s*u[30]/2*(K_sc*Cp_sc*(u[23] - 2*u[37]) - 1)*u[35] - A_s*rho_sc*Cp_sc*K_1*u[30]/2*u[33])
  d(Tp1_otsg)/dt : Fcn  Expr=(u[3]*Cp_p*(u[1] - u[7]) + h_pw*(N*pi*D_it*u[25]/2)*(u[13] - u[7])) / (N*pi*(D_it^2)/4*u[25]/2*rho_p*Cp_p)
  d(Tp2_otsg)/dt : Fcn  Expr=(u[3]*Cp_p*(u[7] - u[8]) + h_pw*(N*pi*D_it*u[25]/2)*(u[14] - u[8])) / (N*pi*(D_it^2)/4*u[25]/2*rho_p*Cp_p)
  d(Tp3_otsg)/dt : Fcn  Expr=(u[3]*Cp_p*(u[8] - u[9]) + h_pw*(N*pi*D_it*u[28]/2)*(u[15] - u[9])) / (N*pi*(D_it^2)/4*u[28]/2*rho_p*Cp_p)
  d(Tp4_otsg)/dt : Fcn  Expr=(u[3]*Cp_p*(u[9] - u[10]) + h_pw*(N*pi*D_it*u[28]/2)*(u[16] - u[10])) / (N*pi*(D_it^2)/4*u[28]/2*rho_p*Cp_p)
  d(Tp5_otsg)/dt : Fcn  Expr=(u[3]*Cp_p*(u[10] - u[11]) + h_pw*(N*pi*D_it*u[30]/2)*(u[17] - u[11])) / (N*pi*(D_it^2)/4*u[30]/2*rho_p*Cp_p)
  d(Tp6_otsg)/dt : Fcn  Expr=(u[3]*Cp_p*(u[11] - u[12]) + h_pw*(N*pi*D_it*u[30]/2)*(u[18] - u[12])) / (N*pi*(D_it^2)/4*u[30]/2*rho_p*Cp_p)
  d(Ts1_otsg)/dt : Fcn  Expr=(h_ws*(N*pi*D_ot*u[25]/2)*(u[13] - u[19]) + u[40]*Cp_s*(u[21] - u[19]) + Cp_s*(u[21] - u[19])*u[38]/2 + (A_s*u[25]/2 - u[39]/2*dHs_dPs)*u[31]) / (u[39]/2*Cp_s)
  d(Ts2_otsg)/dt : Fcn  Expr=(h_ws*(N*pi*D_ot*u[25]/2)*(u[14] - u[21]) + u[42]*Cp_s*(u[37] - u[21]) + (A_s*u[25]/2 - u[39]/2*dHs_dPs)*u[31]) / (u[39]/2*Cp_s)
  d(Tsc2_otsg)/dt : Fcn  Expr=((h_wsc*(N*pi*D_ot*u[30]/2)*(u[18] - u[23]) + Cp_sc*(u[5]*u[2] - (u[5] + u[41])*0.5*u[23]) + A_s*u[30]/2*u[35]) * 2/(A_s*rho_sc*Cp_sc) - u[23]*u[29]) / u[30]
  d(Tw1_otsg)/dt : Fcn  Expr=(h_pw*(N*pi*D_it*u[25]/2)*(u[7] - u[13]) + h_ws*(N*pi*D_ot*u[25]/2)*(u[19] - u[13])) / (N*pi*(D_ot^2 - D_it^2)/4*u[25]/2*rho_w*Cp_w)
  d(Tw2_otsg)/dt : Fcn  Expr=(h_pw*(N*pi*D_it*u[25]/2)*(u[8] - u[14]) + h_ws*(N*pi*D_ot*u[25]/2)*(u[21] - u[14])) / (N*pi*(D_ot^2 - D_it^2)/4*u[25]/2*rho_w*Cp_w)
  d(Tw3_otsg)/dt : Fcn  Expr=(h_pw*(N*pi*D_it*u[28]/2)*(u[9] - u[15]) + h_wb*(N*pi*D_ot*u[28]/2)*(u[37] - u[15])) / (N*pi*(D_ot^2 - D_it^2)/4*u[28]/2*rho_w*Cp_w)
  d(Tw4_otsg)/dt : Fcn  Expr=(h_pw*(N*pi*D_it*u[28]/2)*(u[10] - u[16]) + h_wb*(N*pi*D_ot*u[28]/2)*(u[37] - u[16])) / (N*pi*(D_ot^2 - D_it^2)/4*u[28]/2*rho_w*Cp_w)
  d(Tw5_otsg)/dt : Fcn  Expr=(h_pw*(N*pi*D_it*u[30]/2)*(u[11] - u[17]) + h_wsc*(N*pi*D_ot*u[30]/2)*(u[37] - u[17])) / (N*pi*(D_ot^2 - D_it^2)/4*u[30]/2*rho_w*Cp_w)
  d(Tw6_otsg)/dt : Fcn  Expr=(h_pw*(N*pi*D_it*u[30]/2)*(u[12] - u[18]) + h_wsc*(N*pi*D_ot*u[30]/2)*(u[23] - u[18])) / (N*pi*(D_ot^2 - D_it^2)/4*u[30]/2*rho_w*Cp_w)
  dP_s/dt : Fcn  Expr=(Z_ss*R*(u[38]*(u[19] + u[21]) + u[39]*(u[20] + u[22]))/(2*M_stm) - u[32]*A_s*u[26]) / (A_s*u[25])
  dP_sat/dt : Fcn  Expr=u[31]
  dP_sc/dt : Fcn  Expr=u[31]
  d_M_s/dt : Fcn  Expr=u[42] - u[40]
  rho_b : Fcn  Expr=25.884875705 + 12.835*u[32]
  STEAM TEMPERATURE : Outport
  HITEC OUTLET TEMPERATURE : Outport  Port=2
  STEAM PRESSURE : Outport  Port=3
  STEAM FLOW RATE : Outport  Port=4
  wires:
  FEEDWATER INLET TEMPERATURE/1 -> Mux/2
  d(Tp1_otsg)/dt/1 -> Tp1_otsg/1
  HITEC INLET TEMPERATURE/1 -> Mux/1
  HITEC FLOW RATE/1 -> Mux/3
  HITEC HEAT TRANSFER FRAC/1 -> Mux/4
  PRESSURE SET POINT/1 -> Mux/6
  Tp1_otsg/1 -> Mux/7
  Tp2_otsg/1 -> Mux/8
  d(Tp2_otsg)/dt/1 -> Tp2_otsg/1
  Tp3_otsg/1 -> Mux/9
  d(Tp3_otsg)/dt/1 -> Tp3_otsg/1
  Tp4_otsg/1 -> Mux/10
  d(Tp4_otsg)/dt/1 -> Tp4_otsg/1
  Tp5_otsg/1 -> Mux/11
  d(Tp5_otsg)/dt/1 -> Tp5_otsg/1
  d(Tp6_otsg)/dt/1 -> Tp6_otsg/1
  Tp6_otsg/1 -> HITEC OUTLET TEMPERATURE/1, Mux/12
  Tw1_otsg/1 -> Mux/13
  d(Tw1_otsg)/dt/1 -> Tw1_otsg/1
  d(Tw2_otsg)/dt/1 -> Tw2_otsg/1
  Tw2_otsg/1 -> Mux/14
  Tw3_otsg/1 -> Mux/15
  d(Tw3_otsg)/dt/1 -> Tw3_otsg/1
  d(Tw4_otsg)/dt/1 -> Tw4_otsg/1
  Tw4_otsg/1 -> Mux/16
  Tw5_otsg/1 -> Mux/17
  d(Tw5_otsg)/dt/1 -> Tw5_otsg/1
  d(Tw6_otsg)/dt/1 -> Tw6_otsg/1
  Tw6_otsg/1 -> Mux/18
  Ts1_otsg/1 -> STEAM TEMPERATURE/1, Mux/19
  L_sc/1 -> Mux/30
  L_s/1 -> Unit Delay1/1
  L_b/1 -> Mux/28
  P_s/1 -> Mux/32, STEAM PRESSURE/1
  P_sat/1 -> Mux/34
  P_sc/1 -> Mux/36
  Tsc2_otsg/1 -> Mux/23
  d(Tsc2_otsg)/dt/1 -> Tsc2_otsg/1
  Ts2_otsg/1 -> Mux/21
  rho_b/1 -> Unit Delay/1
  Unit Delay/1 -> Mux/24
  M_s/1 -> Mux/39
  Mux/1 -> W_b/1, W_db/1, d_M_s/dt/1, T_sat/1, dP_sc/dt/1, dP_sat/dt/1, dP_s/dt/1, d(L_sc)/dt/1, d(L_b)/dt/1, d(L_s)/dt/1, L_s/1, rho_b/1, d(Tsc2_otsg)/dt/1, d(Ts2_otsg)/dt/1, d(Ts1_otsg)/dt/1, d(Tw6_otsg)/dt/1, d(Tw5_otsg)/dt/1, d(Tw4_otsg)/dt/1, d(Tw3_otsg)/dt/1, d(Tw2_otsg)/dt/1, d(Tw1_otsg)/dt/1, d(Tp6_otsg)/dt/1, d(Tp5_otsg)/dt/1, d(Tp4_otsg)/dt/1, d(Tp3_otsg)/dt/1, d(Tp2_otsg)/dt/1, d(Tp1_otsg)/dt/1, M_s_fac1/1, Unit Delay4/1
  d(Ts1_otsg)/dt/1 -> Mux/20, Ts1_otsg/1
  d(Ts2_otsg)/dt/1 -> Mux/22, Ts2_otsg/1
  dP_s/dt/1 -> Mux/31, P_s/1
  d(L_b)/dt/1 -> Mux/27, L_b/1
  d(L_s)/dt/1 -> Mux/26
  d(L_sc)/dt/1 -> Mux/29, L_sc/1
  dP_sat/dt/1 -> Mux/33, P_sat/1
  dP_sc/dt/1 -> Mux/35, P_sc/1
  Unit Delay1/1 -> Mux/25
  T_sat/1 -> Mux/37
  M_s_fac1/1 -> Unit Delay2/1
  d_M_s/dt/1 -> Mux/38, M_s/1
  Unit Delay2/1 -> STEAM FLOW RATE/1, Mux/40
  W_db/1 -> Mux/41
  W_b/1 -> Mux/42
  Unit Delay4/1 -> To Workspace/1
  From Workspace1/1 -> PID Controller (2DOF)1/1
  PID Controller (2DOF)1/1 -> Mux/5
  POWER/1 -> PID Controller (2DOF)1/2

== system MSDR_DH_DeplV1sim/SECONDARY SIDE/Variant Subsystem/OTSG ==
  HITEC_INLET : Inport
  POWER LEVEL : Inport  Port=2
  HITEC_FLOW_FRAC : Inport  Port=3
  HITEC_HTC_FRAC : Inport  Port=4
  Clock : Clock
  Clock1 : Clock
  Constant1 : Constant  Value=0
  Constant12 : Constant  Value=T_fw
  Constant13 : Constant  Value=W_p0
  Constant2 : Constant
  Constant4 : Constant  Value=12.5
  Display{12,14..15,47} (4 alike) : Display
  ONCE-THROUGH STEAM GENERATOR : Subsystem
  Product : Product
  SHX TO PHX DELAY1 : VariableTransportDelay  MaximumDelay=1000000000000  InitialOutput=T0_s_shx5(4)
  Scope : Scope
  Switch : Switch  Criteria=u2 > Threshold  Threshold=Trip_UHX
  Switch1 : Switch  Threshold=Trip_UHX
  VAR DELAY FUNC3 : Fcn  Expr=tau_ostg_shx/u
  HITEC_OUTLET : Outport
  wires:
  Constant12/1 -> ONCE-THROUGH STEAM GENERATOR/2(FEEDWATER INLET TEMPERATURE)
  POWER LEVEL/1 -> ONCE-THROUGH STEAM GENERATOR/5(POWER)
  ONCE-THROUGH STEAM GENERATOR/2(HITEC OUTLET TEMPERATURE) -> Display47/1, Switch/3
  Clock/1 -> Switch/2
  Switch/1 -> HITEC_OUTLET/1, Scope/1
  Constant13/1 -> Product/2
  HITEC_FLOW_FRAC/1 -> Product/1, [HITEC_FLOW_FRAC]
  VAR DELAY FUNC3/1 -> SHX TO PHX DELAY1/2
  Product/1 -> ONCE-THROUGH STEAM GENERATOR/3(HITEC FLOW RATE)
  Clock1/1 -> Switch1/2
  HITEC_HTC_FRAC/1 -> ONCE-THROUGH STEAM GENERATOR/4(HITEC HEAT TRANSFER FRAC)
  Switch1/1 -> ONCE-THROUGH STEAM GENERATOR/Enable
  SHX TO PHX DELAY1/1 -> Switch/1
  [HITEC_IN_TEMP] -> SHX TO PHX DELAY1/1
  [HITEC_FLOW_FRAC] -> VAR DELAY FUNC3/1
  ONCE-THROUGH STEAM GENERATOR/3(STEAM PRESSURE) -> Display14/1
  Constant4/1 -> ONCE-THROUGH STEAM GENERATOR/6(PRESSURE SET POINT)
  ONCE-THROUGH STEAM GENERATOR/4(STEAM FLOW RATE) -> Display15/1
  Constant2/1 -> Switch1/3
  ONCE-THROUGH STEAM GENERATOR/1(STEAM TEMPERATURE) -> Display12/1
  HITEC_INLET/1 -> ONCE-THROUGH STEAM GENERATOR/1(HITEC INLET TEMPERATURE), [HITEC_IN_TEMP]
  Constant1/1 -> Switch1/1

== system MSDR_DH_DeplV1sim/SECONDARY SIDE/Variant Subsystem/UHX ==
  HITEC_INLET : Inport
  HITEC_FLOW_FRAC : Inport  Port=2
  Clock : Clock
  Clock1 : Clock
  Constant1 : Constant  Value=0
  Constant2 : Constant
  SHX TO PHX DELAY1 : VariableTransportDelay  MaximumDelay=1000000000000  InitialOutput=T0_s_shx5(4)
  Scope : Scope
  Switch : Switch  Criteria=u2 > Threshold  Threshold=Trip_UHX
  Switch1 : Switch  Threshold=Trip_UHX
  UHX : Subsystem
  VAR DELAY FUNC3 : Fcn  Expr=tau_ostg_shx/u
  HITEC_OUTLET : Outport
  wires:
  HITEC_FLOW_FRAC/1 -> [HITEC_FLOW_FRAC], UHX/2(HITEC_FLOW_FRAC)
  HITEC_INLET/1 -> [HITEC_IN_TEMP], UHX/1(HITEC_INLET)
  Switch/1 -> Scope/1, HITEC_OUTLET/1
  Clock/1 -> Switch/2
  [HITEC_FLOW_FRAC] -> VAR DELAY FUNC3/1
  UHX/1(HITEC_OUTLET) -> Switch/3
  VAR DELAY FUNC3/1 -> SHX TO PHX DELAY1/2
  SHX TO PHX DELAY1/1 -> Switch/1
  [HITEC_IN_TEMP] -> SHX TO PHX DELAY1/1
  Constant1/1 -> Switch1/1
  Constant2/1 -> Switch1/3
  Switch1/1 -> UHX/Enable
  Clock1/1 -> Switch1/2

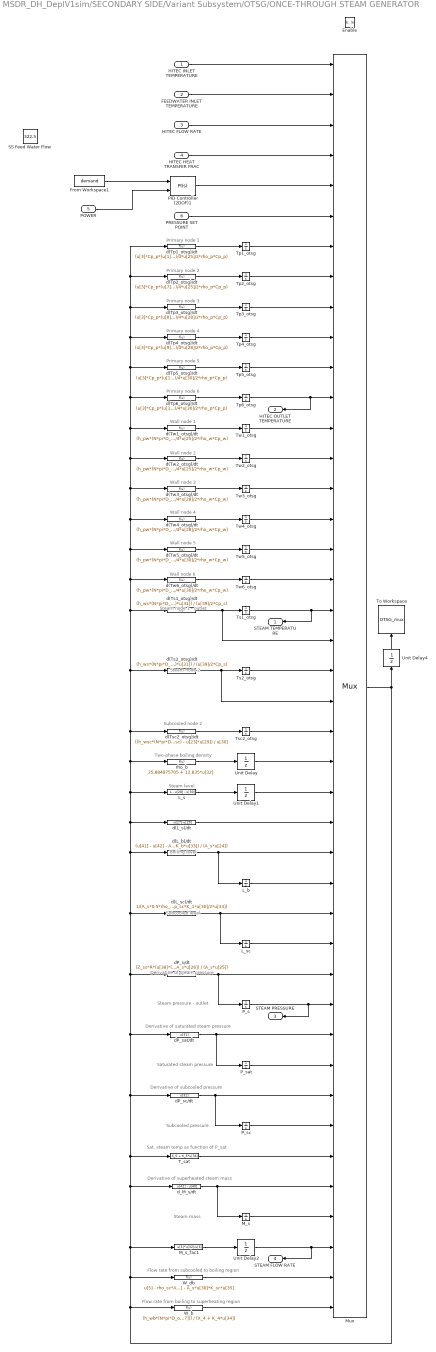
== system MSDR_DH_DeplV1sim/SECONDARY SIDE/Variant Subsystem/OTSG/ONCE-THROUGH STEAM GENERATOR ==
  note: Primary node 1
  note: Primary node 2
  note: Primary node 3
  note: Primary node 4
  note: Primary node 5
  note: Primary node 6
  note: Wall node 1
  note: Wall node 2
  note: Wall node 3
  note: Wall node 4
  note: Wall node 5
  note: Wall node 6
  note: Steam node 1 - outlet
  note: Steam level
  note: Boiling level
  note: Subcooled level
  note: Derivative of saturated steam pressure
  note: Sat. steam temp as function of P_sat
  note: Saturated steam pressure
  note: Subcooled pressure
  note: Derivative of steam pressure
  note: Derivative of subcooled pressure
  note: Steam pressure - outlet
  note: Subcooled node 2
  note: Steam node 2
  note: Two-phase boiling density
  note: Derivative of superheated steam mass
  note: Steam mass
  note: Flow rate from subcooled to boiling region
  note: Flow rate from boiling to superheating region
  HITEC INLET TEMPERATURE : Inport
  FEEDWATER INLET TEMPERATURE : Inport  Port=2
  HITEC FLOW RATE : Inport  Port=3
  HITEC HEAT TRANSFER FRAC : Inport  Port=4
  POWER : Inport  Port=5
  PRESSURE SET POINT : Inport  Port=6
  Enable : EnablePort
  From Workspace1 : FromWorkspace  VariableName=demand  SampleTime=1  Interpolate=off  OutputAfterFinalValue=Holding final value
  L_b : Integrator  InitialCondition=L_b
  L_s : Fcn  Expr=L - u[28] - u[30]
  L_sc : Integrator  InitialCondition=.5344
  M_s : Integrator  InitialCondition=A_s*rho_s*L_s
  M_s_fac1 : Fcn  Expr=u[5]*u[32]/u[6]
  Mux : Mux  Inputs=42
      settings: DisplayOption=signals
  PID Controller (2DOF)1 : simulink/Continuous/PID Controller (2DOF)  Controller=PI  Form=Parallel  TimeDomain=Continuous-time  SampleTime=-1  IntegratorMethod=Forward Euler  FilterMethod=Forward Euler  ControllerParametersSource=internal  P=250  I=5  D=1  UseFilter=on  N=100  b=1  c=1  TunerSelectOption=Transfer Function Based (PID Tuner App)  InitialConditionSource=internal  InitialConditionForIntegrator=0  InitialConditionForFilter=0  DifferentiatorICPrevScaledInput=0  ExternalReset=none  TrackingMode=off  Kt=1  LimitOutput=on  UpperSaturationLimit=1000000  LowerSaturationLimit=1  LinearizeAsGain=on  AntiWindupMode=none  Kb=1  POutMin=[]  POutMax=[]  IOutMin=[]  IOutMax=[]  DOutMin=[]  DOutMax=[]  NOutMin=[]  NOutMax=[]  bOutMin=[]  bOutMax=[]  cOutMin=[]  cOutMax=[]  SumOutMin=[]  SumOutMax=[]  SaturationOutMin=[]  SaturationOutMax=[]  PParamMin=[]  PParamMax=[]  IParamMin=[]  IParamMax=[]  DParamMin=[]  DParamMax=[]  NParamMin=[]  NParamMax=[]  bParamMin=[]  bParamMax=[]  cParamMin=[]  cParamMax=[]  KbParamMin=[]  KbParamMax=[]  KtParamMin=[]  KtParamMax=[]  KbOutMin=[]  KbOutMax=[]  KtOutMin=[]  KtOutMax=[]  IntegratorOutMin=[]  IntegratorOutMax=[]  FilterOutMin=[]  FilterOutMax=[]  SumI1OutMin=[]  SumI1OutMax=[]  SumI2OutMin=[]  SumI2OutMax=[]  SumI3OutMin=[]  SumI3OutMax=[]  SumI4OutMin=[]  SumI4OutMax=[]  SumDOutMin=[]  SumDOutMax=[]  Sum1OutMin=[]  Sum1OutMax=[]  Sum2OutMin=[]  Sum2OutMax=[]  Sum3OutMin=[]  Sum3OutMax=[]  DifferentiatorOutMin=[]  DifferentiatorOutMax=[]  FilterDiffOutCoefMin=[]  FilterDiffOutCoefMax=[]  ReciprocalOutMin=[]  ReciprocalOutMax=[]  SumDenOutMin=[]  SumDenOutMax=[]  SumNumOutMin=[]  SumNumOutMax=[]  DivideOutMin=[]  DivideOutMax=[]  IntegratorContinuousStateAttributes=''  IntegratorStateMustResolveToSignalObject=off  IntegratorRTWStateStorageClass=Auto  FilterContinuousStateAttributes=''  FilterStateMustResolveToSignalObject=off  FilterRTWStateStorageClass=Auto  ParallelPVariant=InternalParameters  IdealPVariant=Disabled  IVariant=InternalParameters  DVariant=Disabled  bVariant=InternalParameters  cVariant=Disabled  IntegratorVariant=Continuous  SatVariant=Enabled  AWVariant=Passthrough  PCopyVariant=Disabled  TRVariant=Disabled  FdbkBlocksVariant=Forward  IdealPFdbkVariant=Disabled  SatFdbkVariant=Disabled  DerivativeFilterVariant=Disabled  NVariant=Disabled  NCopyVariant=Disabled_SignalSpec  FilterICVariant=Disabled  IntegratorICVariant=InternalICs  ExternalResetVariant=Disabled  TRSumVariant=Passthrough  SumFdbkVariant=Disabled  SumVariant=Sum_PI
  P_s : Integrator  InitialCondition=P_s
  P_sat : Integrator  InitialCondition=P_sat
  P_sc : Integrator  InitialCondition=P_sc
  SS Feed Water Flow : Constant  Value=322.5
  T_sat : Fcn  Expr=X_5 + K_5*u[34]
  To Workspace : ToWorkspace  VariableName=OTSG_mux  SaveFormat=Timeseries  SampleTime=-1
  Tp1_otsg : Integrator  InitialCondition=T_p1
  Tp2_otsg : Integrator  InitialCondition=T_p2
  Tp3_otsg : Integrator  InitialCondition=T_p3
  Tp4_otsg : Integrator  InitialCondition=T_p4
  Tp5_otsg : Integrator  InitialCondition=T_p5
  Tp6_otsg : Integrator  InitialCondition=T_p6
  Ts1_otsg : Integrator  InitialCondition=T_s1
  Ts2_otsg : Integrator  InitialCondition=T_s2
  Tsc2_otsg : Integrator  InitialCondition=T_sc2
  Tw1_otsg : Integrator  InitialCondition=T_w1
  Tw2_otsg : Integrator  InitialCondition=T_w2
  Tw3_otsg : Integrator  InitialCondition=T_w3
  Tw4_otsg : Integrator  InitialCondition=T_w4
  Tw5_otsg : Integrator  InitialCondition=T_w5
  Tw6_otsg : Integrator  InitialCondition=T_w6
  Unit Delay : UnitDelay  InitialCondition=rho_b  SampleTime=-1  HasFrameUpgradeWarning=on
  Unit Delay1 : UnitDelay  InitialCondition=L_s  SampleTime=-1  HasFrameUpgradeWarning=on
  Unit Delay2 : UnitDelay  InitialCondition=W_fw  SampleTime=-1  HasFrameUpgradeWarning=on
  Unit Delay4 : UnitDelay  SampleTime=-1  HasFrameUpgradeWarning=on
  W_b : Fcn  Expr=(h_wb*(N*pi*D_ot*u[28])*(0.5*u[15] + 0.5*u[16] - u[37])) / (X_4 + K_4*u[34])
  W_db : Fcn  Expr=u[5] - rho_sc*A_s*u[29] - A_s*u[30]*K_sc*u[35]
  d(L_b)/dt : Fcn  Expr=(u[41] - u[42] - A_s*u[28]*K_b*u[33]) / (A_s*u[24])
  d(L_s)/dt : Fcn  Expr=-u[27]-u[29]
  d(L_sc)/dt : Fcn  Expr=1/(A_s*0.5*rho_sc*Cp_sc*(u[23] - u[37])) * (h_wsc*N*pi*D_ot*u[30]/2*(u[17] - u[37]) + Cp_sc*(u[5]*u[23] - (u[5] + u[41])*0.5*u[37]) - A_s*u[30]/2*(K_sc*Cp_sc*(u[23] - 2*u[37]) - 1)*u[35] - A_s*rho_sc*Cp_sc*K_1*u[30]/2*u[33])
  d(Tp1_otsg)/dt : Fcn  Expr=(u[3]*Cp_p*(u[1] - u[7]) + h_pw*(N*pi*D_it*u[25]/2)*(u[13] - u[7])) / (N*pi*(D_it^2)/4*u[25]/2*rho_p*Cp_p)
  d(Tp2_otsg)/dt : Fcn  Expr=(u[3]*Cp_p*(u[7] - u[8]) + h_pw*(N*pi*D_it*u[25]/2)*(u[14] - u[8])) / (N*pi*(D_it^2)/4*u[25]/2*rho_p*Cp_p)
  d(Tp3_otsg)/dt : Fcn  Expr=(u[3]*Cp_p*(u[8] - u[9]) + h_pw*(N*pi*D_it*u[28]/2)*(u[15] - u[9])) / (N*pi*(D_it^2)/4*u[28]/2*rho_p*Cp_p)
  d(Tp4_otsg)/dt : Fcn  Expr=(u[3]*Cp_p*(u[9] - u[10]) + h_pw*(N*pi*D_it*u[28]/2)*(u[16] - u[10])) / (N*pi*(D_it^2)/4*u[28]/2*rho_p*Cp_p)
  d(Tp5_otsg)/dt : Fcn  Expr=(u[3]*Cp_p*(u[10] - u[11]) + h_pw*(N*pi*D_it*u[30]/2)*(u[17] - u[11])) / (N*pi*(D_it^2)/4*u[30]/2*rho_p*Cp_p)
  d(Tp6_otsg)/dt : Fcn  Expr=(u[3]*Cp_p*(u[11] - u[12]) + h_pw*(N*pi*D_it*u[30]/2)*(u[18] - u[12])) / (N*pi*(D_it^2)/4*u[30]/2*rho_p*Cp_p)
  d(Ts1_otsg)/dt : Fcn  Expr=(h_ws*(N*pi*D_ot*u[25]/2)*(u[13] - u[19]) + u[40]*Cp_s*(u[21] - u[19]) + Cp_s*(u[21] - u[19])*u[38]/2 + (A_s*u[25]/2 - u[39]/2*dHs_dPs)*u[31]) / (u[39]/2*Cp_s)
  d(Ts2_otsg)/dt : Fcn  Expr=(h_ws*(N*pi*D_ot*u[25]/2)*(u[14] - u[21]) + u[42]*Cp_s*(u[37] - u[21]) + (A_s*u[25]/2 - u[39]/2*dHs_dPs)*u[31]) / (u[39]/2*Cp_s)
  d(Tsc2_otsg)/dt : Fcn  Expr=((h_wsc*(N*pi*D_ot*u[30]/2)*(u[18] - u[23]) + Cp_sc*(u[5]*u[2] - (u[5] + u[41])*0.5*u[23]) + A_s*u[30]/2*u[35]) * 2/(A_s*rho_sc*Cp_sc) - u[23]*u[29]) / u[30]
  d(Tw1_otsg)/dt : Fcn  Expr=(h_pw*(N*pi*D_it*u[25]/2)*(u[7] - u[13]) + h_ws*(N*pi*D_ot*u[25]/2)*(u[19] - u[13])) / (N*pi*(D_ot^2 - D_it^2)/4*u[25]/2*rho_w*Cp_w)
  d(Tw2_otsg)/dt : Fcn  Expr=(h_pw*(N*pi*D_it*u[25]/2)*(u[8] - u[14]) + h_ws*(N*pi*D_ot*u[25]/2)*(u[21] - u[14])) / (N*pi*(D_ot^2 - D_it^2)/4*u[25]/2*rho_w*Cp_w)
  d(Tw3_otsg)/dt : Fcn  Expr=(h_pw*(N*pi*D_it*u[28]/2)*(u[9] - u[15]) + h_wb*(N*pi*D_ot*u[28]/2)*(u[37] - u[15])) / (N*pi*(D_ot^2 - D_it^2)/4*u[28]/2*rho_w*Cp_w)
  d(Tw4_otsg)/dt : Fcn  Expr=(h_pw*(N*pi*D_it*u[28]/2)*(u[10] - u[16]) + h_wb*(N*pi*D_ot*u[28]/2)*(u[37] - u[16])) / (N*pi*(D_ot^2 - D_it^2)/4*u[28]/2*rho_w*Cp_w)
  d(Tw5_otsg)/dt : Fcn  Expr=(h_pw*(N*pi*D_it*u[30]/2)*(u[11] - u[17]) + h_wsc*(N*pi*D_ot*u[30]/2)*(u[37] - u[17])) / (N*pi*(D_ot^2 - D_it^2)/4*u[30]/2*rho_w*Cp_w)
  d(Tw6_otsg)/dt : Fcn  Expr=(h_pw*(N*pi*D_it*u[30]/2)*(u[12] - u[18]) + h_wsc*(N*pi*D_ot*u[30]/2)*(u[23] - u[18])) / (N*pi*(D_ot^2 - D_it^2)/4*u[30]/2*rho_w*Cp_w)
  dP_s/dt : Fcn  Expr=(Z_ss*R*(u[38]*(u[19] + u[21]) + u[39]*(u[20] + u[22]))/(2*M_stm) - u[32]*A_s*u[26]) / (A_s*u[25])
  dP_sat/dt : Fcn  Expr=u[31]
  dP_sc/dt : Fcn  Expr=u[31]
  d_M_s/dt : Fcn  Expr=u[42] - u[40]
  rho_b : Fcn  Expr=25.884875705 + 12.835*u[32]
  STEAM TEMPERATURE : Outport
  HITEC OUTLET TEMPERATURE : Outport  Port=2
  STEAM PRESSURE : Outport  Port=3
  STEAM FLOW RATE : Outport  Port=4
  wires:
  FEEDWATER INLET TEMPERATURE/1 -> Mux/2
  d(Tp1_otsg)/dt/1 -> Tp1_otsg/1
  HITEC INLET TEMPERATURE/1 -> Mux/1
  HITEC FLOW RATE/1 -> Mux/3
  HITEC HEAT TRANSFER FRAC/1 -> Mux/4
  PRESSURE SET POINT/1 -> Mux/6
  Tp1_otsg/1 -> Mux/7
  Tp2_otsg/1 -> Mux/8
  d(Tp2_otsg)/dt/1 -> Tp2_otsg/1
  Tp3_otsg/1 -> Mux/9
  d(Tp3_otsg)/dt/1 -> Tp3_otsg/1
  Tp4_otsg/1 -> Mux/10
  d(Tp4_otsg)/dt/1 -> Tp4_otsg/1
  Tp5_otsg/1 -> Mux/11
  d(Tp5_otsg)/dt/1 -> Tp5_otsg/1
  d(Tp6_otsg)/dt/1 -> Tp6_otsg/1
  Tp6_otsg/1 -> HITEC OUTLET TEMPERATURE/1, Mux/12
  Tw1_otsg/1 -> Mux/13
  d(Tw1_otsg)/dt/1 -> Tw1_otsg/1
  d(Tw2_otsg)/dt/1 -> Tw2_otsg/1
  Tw2_otsg/1 -> Mux/14
  Tw3_otsg/1 -> Mux/15
  d(Tw3_otsg)/dt/1 -> Tw3_otsg/1
  d(Tw4_otsg)/dt/1 -> Tw4_otsg/1
  Tw4_otsg/1 -> Mux/16
  Tw5_otsg/1 -> Mux/17
  d(Tw5_otsg)/dt/1 -> Tw5_otsg/1
  d(Tw6_otsg)/dt/1 -> Tw6_otsg/1
  Tw6_otsg/1 -> Mux/18
  Ts1_otsg/1 -> STEAM TEMPERATURE/1, Mux/19
  L_sc/1 -> Mux/30
  L_s/1 -> Unit Delay1/1
  L_b/1 -> Mux/28
  P_s/1 -> Mux/32, STEAM PRESSURE/1
  P_sat/1 -> Mux/34
  P_sc/1 -> Mux/36
  Tsc2_otsg/1 -> Mux/23
  d(Tsc2_otsg)/dt/1 -> Tsc2_otsg/1
  Ts2_otsg/1 -> Mux/21
  rho_b/1 -> Unit Delay/1
  Unit Delay/1 -> Mux/24
  M_s/1 -> Mux/39
  Mux/1 -> W_b/1, W_db/1, d_M_s/dt/1, T_sat/1, dP_sc/dt/1, dP_sat/dt/1, dP_s/dt/1, d(L_sc)/dt/1, d(L_b)/dt/1, d(L_s)/dt/1, L_s/1, rho_b/1, d(Tsc2_otsg)/dt/1, d(Ts2_otsg)/dt/1, d(Ts1_otsg)/dt/1, d(Tw6_otsg)/dt/1, d(Tw5_otsg)/dt/1, d(Tw4_otsg)/dt/1, d(Tw3_otsg)/dt/1, d(Tw2_otsg)/dt/1, d(Tw1_otsg)/dt/1, d(Tp6_otsg)/dt/1, d(Tp5_otsg)/dt/1, d(Tp4_otsg)/dt/1, d(Tp3_otsg)/dt/1, d(Tp2_otsg)/dt/1, d(Tp1_otsg)/dt/1, M_s_fac1/1, Unit Delay4/1
  d(Ts1_otsg)/dt/1 -> Mux/20, Ts1_otsg/1
  d(Ts2_otsg)/dt/1 -> Mux/22, Ts2_otsg/1
  dP_s/dt/1 -> Mux/31, P_s/1
  d(L_b)/dt/1 -> Mux/27, L_b/1
  d(L_s)/dt/1 -> Mux/26
  d(L_sc)/dt/1 -> Mux/29, L_sc/1
  dP_sat/dt/1 -> Mux/33, P_sat/1
  dP_sc/dt/1 -> Mux/35, P_sc/1
  Unit Delay1/1 -> Mux/25
  T_sat/1 -> Mux/37
  M_s_fac1/1 -> Unit Delay2/1
  d_M_s/dt/1 -> Mux/38, M_s/1
  Unit Delay2/1 -> STEAM FLOW RATE/1, Mux/40
  W_db/1 -> Mux/41
  W_b/1 -> Mux/42
  Unit Delay4/1 -> To Workspace/1
  From Workspace1/1 -> PID Controller (2DOF)1/1
  PID Controller (2DOF)1/1 -> Mux/5
  POWER/1 -> PID Controller (2DOF)1/2
